simulink model "p2"  (R2021a)
settings: Solver=FixedStepAuto  StartTime=0.0  StopTime=inf  RelTol=1e-3
settings Model: EnablePacing=on  Creator=Abbas  LastModifiedBy=smrh1

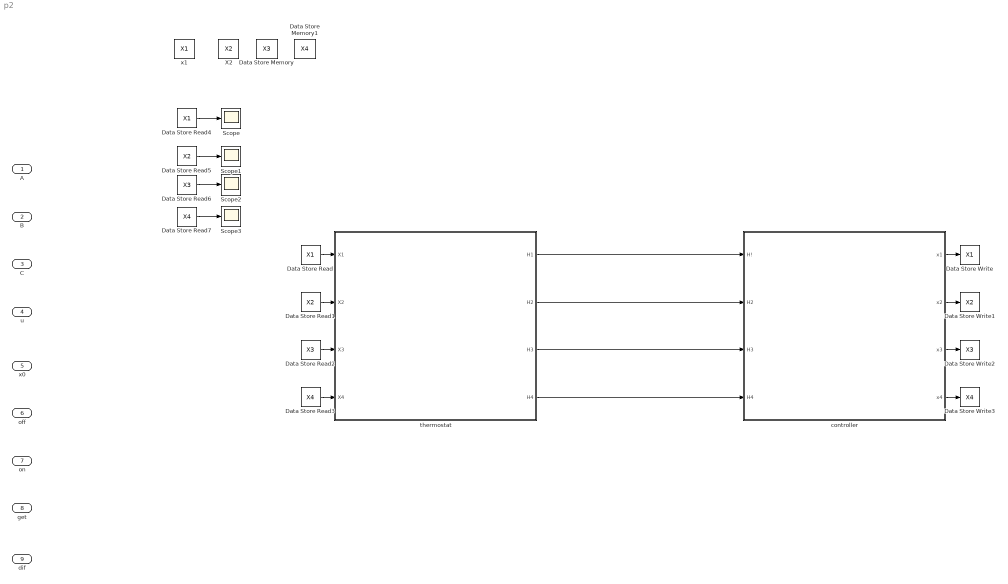
== system p2 ==
  A : Inport
  B : Inport  Port=2
  C : Inport  Port=3
  u : Inport  Port=4
  x0 : Inport  Port=5
  off : Inport  Port=6
  on : Inport  Port=7
  get : Inport  Port=8
  dif : Inport  Port=9
  Data Store Memory : DataStoreMemory  DataStoreName=X3  ReadBeforeWriteMsg=warning  WriteAfterWriteMsg=warning  WriteAfterReadMsg=warning  InitialValue=16.5  ShowAdditionalParam=off
  Data Store Memory1 : DataStoreMemory  DataStoreName=X4  ReadBeforeWriteMsg=warning  WriteAfterWriteMsg=warning  WriteAfterReadMsg=warning  InitialValue=16.5  ShowAdditionalParam=off
  Data Store Read : DataStoreRead  DataStoreName=X1  IndexOptions=Index vector (dialog)  Indices=1  OutputSizes=1
  Data Store Read1 : DataStoreRead  DataStoreName=X2  IndexOptions=Index vector (dialog)  Indices=1  OutputSizes=1
  Data Store Read2 : DataStoreRead  DataStoreName=X3  IndexOptions=Index vector (dialog)  Indices=1  OutputSizes=1
  Data Store Read3 : DataStoreRead  DataStoreName=X4  IndexOptions=Index vector (dialog)  Indices=1  OutputSizes=1
  Data Store Read4 : DataStoreRead  DataStoreName=X1  IndexOptions=Index vector (dialog)  Indices=1  OutputSizes=1
  Data Store Read5 : DataStoreRead  DataStoreName=X2  IndexOptions=Index vector (dialog)  Indices=1  OutputSizes=1
  Data Store Read6 : DataStoreRead  DataStoreName=X3  IndexOptions=Index vector (dialog)  Indices=1  OutputSizes=1
  Data Store Read7 : DataStoreRead  DataStoreName=X4  IndexOptions=Index vector (dialog)  Indices=1  OutputSizes=1
  Data Store Write : DataStoreWrite  DataStoreName=X1  IndexOptions=Index vector (dialog)  Indices=1  OutputSizes=1
  Data Store Write1 : DataStoreWrite  DataStoreName=X2  IndexOptions=Index vector (dialog)  Indices=1  OutputSizes=1
  Data Store Write2 : DataStoreWrite  DataStoreName=X3  IndexOptions=Index vector (dialog)  Indices=1  OutputSizes=1
  Data Store Write3 : DataStoreWrite  DataStoreName=X4  IndexOptions=Index vector (dialog)  Indices=1  OutputSizes=1
  Scope{,1..3} (4 alike) : Scope
  X2 : DataStoreMemory  DataStoreName=X2  ReadBeforeWriteMsg=warning  WriteAfterWriteMsg=warning  WriteAfterReadMsg=warning  InitialValue=16.5  ShowAdditionalParam=off
  controller : Subsystem
  thermostat : Subsystem
  x1 : DataStoreMemory  DataStoreName=X1  ReadBeforeWriteMsg=warning  WriteAfterWriteMsg=warning  WriteAfterReadMsg=warning  InitialValue=16.5  ShowAdditionalParam=off
  wires:
  thermostat/4(H4) -> controller/4(H4)
  thermostat/3(H3) -> controller/3(H3)
  thermostat/2(H2) -> controller/2(H2)
  thermostat/1(H1) -> controller/1(H!)
  controller/1(x1) -> Data Store Write/1
  Data Store Read/1 -> thermostat/1(X1)
  Data Store Read1/1 -> thermostat/2(X2)
  Data Store Read2/1 -> thermostat/3(X3)
  Data Store Read3/1 -> thermostat/4(X4)
  controller/2(x2) -> Data Store Write1/1
  controller/3(x3) -> Data Store Write2/1
  controller/4(x4) -> Data Store Write3/1
  Data Store Read4/1 -> Scope/1
  Data Store Read5/1 -> Scope1/1
  Data Store Read6/1 -> Scope2/1
  Data Store Read7/1 -> Scope3/1

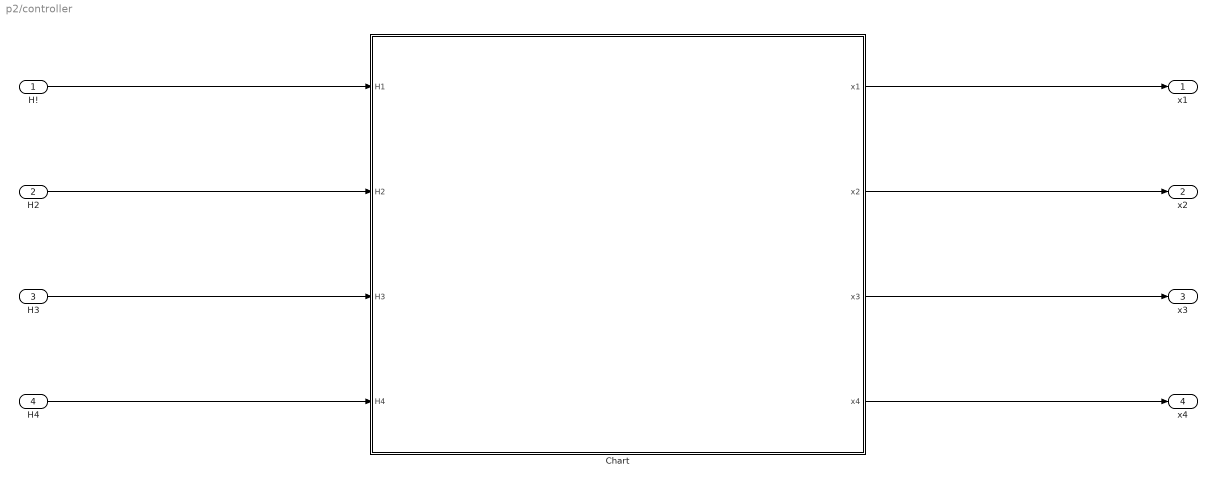
== system p2/controller ==
  H! : Inport
  H2 : Inport  Port=2
  H3 : Inport  Port=3
  H4 : Inport  Port=4
  Chart : Stateflow chart  TreatAsAtomicUnit=on
  x1 : Outport
  x2 : Outport  Port=2
  x3 : Outport  Port=3
  x4 : Outport  Port=4
  wires:
  Chart/1(x1) -> x1/1
  Chart/2(x2) -> x2/1
  Chart/3(x3) -> x3/1
  Chart/4(x4) -> x4/1
  H!/1 -> Chart/1(H1)
  H2/1 -> Chart/2(H2)
  H3/1 -> Chart/3(H3)
  H4/1 -> Chart/4(H4)

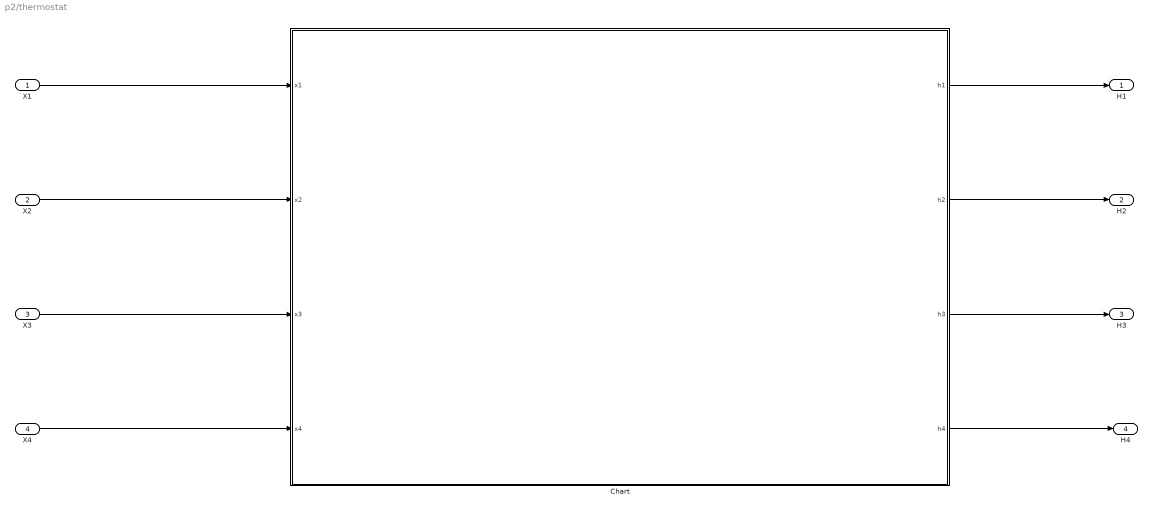
== system p2/thermostat ==
  X1 : Inport
  X2 : Inport  Port=2
  X3 : Inport  Port=3
  X4 : Inport  Port=4
  Chart : Stateflow chart  TreatAsAtomicUnit=on
  H1 : Outport
  H2 : Outport  Port=2
  H3 : Outport  Port=3
  H4 : Outport  Port=4
  wires:
  Chart/1(h1) -> H1/1
  Chart/2(h2) -> H2/1
  Chart/3(h3) -> H3/1
  Chart/4(h4) -> H4/1
  X2/1 -> Chart/2(x2)
  X4/1 -> Chart/4(x4)
  X3/1 -> Chart/3(x3)
  X1/1 -> Chart/1(x1)

== stateflow chart p2/thermostat/Chart ==
  state st13
    du:
    h2 = 0;
    h4 = 0;
    state s1 [parallel]
      settings: executionOrder=1
      state s1_on
        du:
        h1 = 1
      state s1_off
        du:
        h1 = 0
      st13.s1.s1_on -> ? : [x1>=off1& after(1,sec)]
      st13.s1.s1_off -> st13.s1.s1_on : [x1<=on1& after(1,sec)]
      (default) -> st13.s1.s1_off
    state s2 [parallel]
      settings: executionOrder=2
      state s3_on
        du:
        h3 = 1
      state s3_off
        du:
        h3 = 0
      st13.s2.s3_on -> ? : [x3>=off3& after(1,sec)]
      st13.s2.s3_off -> st13.s2.s3_on : [x3<=on3& after(1,sec)]
      (default) -> st13.s2.s3_off
  state st14
    du:
    h2 = 0;
    h3 = 0;
    state s1 [parallel]
      settings: executionOrder=1
      state s1_on
        du:
        h1 = 1
      state s1_off
        du:
        h1 = 0
      st14.s1.s1_on -> ? : [x1>=off1& after(1,sec)]
      st14.s1.s1_off -> st14.s1.s1_on : [x1<=on1& after(1,sec)]
      (default) -> st14.s1.s1_off
    state s4 [parallel]
      settings: executionOrder=2
      state s4_on
        du:
        h4 = 1
      state s4_off
        du:
        h4 = 0
      st14.s4.s4_on -> ? : [x4>=off4& after(1,sec)]
      st14.s4.s4_off -> st14.s4.s4_on : [x4<=on4& after(1,sec)]
      (default) -> st14.s4.s4_off
  state st12
    du:
    h3 = 0;
    h4 = 0;
    state s1 [parallel]
      settings: executionOrder=1
      state s1_on1
        du:
        h1 = 1
      state s1_off
        du:
        h1 = 0
      s1_on1 -> ? : [x1>=off1 & after(1,sec)]
      st12.s1.s1_off -> s1_on1 : [x1<=on1 & after(1,sec)]
      (default) -> st12.s1.s1_off
    state s2 [parallel]
      settings: executionOrder=2
      state s2_on
        du:
        h2 = 1
      state s1_off1
        du:
        h2 = 0
      st12.s2.s2_on -> ? : [x2>=off2 & after(1,sec)]
      s1_off1 -> st12.s2.s2_on : [x2<=on2 & after(1,sec)]
      (default) -> s1_off1
  state st24
    du:
    h1 = 0;
    h3 = 0;
    state s2 [parallel]
      settings: executionOrder=1
      state s2_on
        du:
        h2 = 1
      state s2_off
        du:
        h2 = 0
      st24.s2.s2_on -> ? : [x2>=off2& after(1,sec)]
      s2_off -> st24.s2.s2_on : [x2<=on2& after(1,sec)]
      (default) -> s2_off
    state s4 [parallel]
      settings: executionOrder=2
      state s4_on
        du:
        h4 = 1
      state s4_off
        du:
        h4 = 0
      st24.s4.s4_on -> ? : [x4>=off4& after(1,sec)]
      st24.s4.s4_off -> st24.s4.s4_on : [x4<=on4& after(1,sec)]
      (default) -> st24.s4.s4_off
  state st34
    du:
    h1 = 0;
    h2 = 0;
    state s3 [parallel]
      settings: executionOrder=1
      state s3_on
        du:
        h3 = 1
      state s3_off
        du:
        h3 = 0
      st34.s3.s3_on -> ? : [x1>=off1& after(1,sec)]
      st34.s3.s3_off -> st34.s3.s3_on : [x1<=on1& after(1,sec)]
      (default) -> st34.s3.s3_off
    state s4 [parallel]
      settings: executionOrder=2
      state s4_on
        du:
        h4 = 1
      state s4_off
        du:
        h4 = 0
      st34.s4.s4_on -> ? : [x4>=off4& after(1,sec)]
      st34.s4.s4_off -> st34.s4.s4_on : [x4<=on4& after(1,sec)]
      (default) -> st34.s4.s4_off
  state st23
    du:
    h1 = 0;
    h4 = 0;
    state s2 [parallel]
      settings: executionOrder=1
      state s2_on
        du:
        h2 = 1
      state s1_off
        du:
        h2 = 0
      (default) -> st23.s2.s2_on
      st23.s2.s2_on -> ? : [x2>=off2 & after(1,sec)]
      st23.s2.s1_off -> st23.s2.s2_on : [x2<=on2& after(1,sec)]
    state s3 [parallel]
      settings: executionOrder=2
      state s3_on
        du:
        h3 = 1
      state s3_off
        du:
        h3 = 0
      (default) -> st23.s3.s3_on
      st23.s3.s3_on -> ? : [x3>=off3& after(1,sec)]
      st23.s3.s3_off -> st23.s3.s3_on : [x3<=on3 & after(1,sec)]
  state start
  st12 -> st13 [order 1] : [x2-x3>=dif3 & x3<=get3]
  st13 -> st14 [order 2] : [x3-x4>=dif4 & x4<=get4]
  st13 -> st12 [order 1] : [x3-x2>=dif2 & x2<=get2]
  st14 -> st13 [order 2] : [x4-x3>=dif3 & x3<=get3]
  st13 -> st34 [order 5] : [x1-x4>=dif4 & x4<=get4]
  st34 -> st13 [order 2] : [x4-x1>=dif1 & x1<=get1]
  st13 -> st23 [order 3] : [(x1-x2>=dif2 & x2<=get2)]
  st23 -> st14 [order 3] : [((x2-x4>=dif4 & x4<=get4) & (x3-x1>=dif1 & x1<=get1)) | ((x3-x4>=dif4 & x4<=get4) & (x2-x1>=dif1 & x1<=get1))]
  st23 -> st13 [order 2] : [(x2-x1>=dif1 & x1<=get1)]
  st14 -> st23 [order 3] : [((x4-x2>=dif2 & x2<=get2) & (x1-x3>=dif3 & x3<=get3)) |((x1-x2>=dif2 & x2<=get2) & (x4-x3>=dif3 & x3<=get3))]
  st12 -> st14 [order 3] : [x2-x4>=dif4 & x4<=get4]
  st14 -> st12 [order 1] : [x4-x2>=dif2 & x2<=get2]
  st12 -> st34 [order 5] : [((x1-x4>=dif4 & x4<=get4) & (x2-x3>=dif3 & x3<=get3)) | ((x2-x4>=dif4 & x4<=get4) & (x1-x3>=dif3 & x3<=get3))]
  st34 -> st12 [order 1] : [((x4-x1>=dif1 & x1<=get1) & (x3-x2>=dif2 & x2<=get2)) | ((x2-x4>=dif4 & x4<=get4) & (x1-x3>=dif3 & x3<=get3))]
  st14 -> st34 [order 5] : [x1-x3>=dif3 & x3<=get3]
  st34 -> st14 [order 3] : [x3-x1>=dif1 & x1<=get1]
  st13 -> st24 [order 4] : [((x1-x2>=dif2 & x2<=get2) & (x3-x4>=dif4 & x4<=get4)) | ((x3-x2>=dif2 & x2<=get2) & (x1-x4>=dif4 & x4<=get4))]
  st24 -> st13 [order 2] : [((x2-x1>=dif1 & x1<=get1) & (x4-x3>=dif3 & x3<=get3)) | ((x4-x1>=dif1 & x1<=get1) & (x2-x3>=dif3 & x3<=get3))]
  st24 -> st14 [order 3] : [x2-x4>=dif4 & x4<=get4]
  st14 -> st24 [order 4] : [x4-x2>=dif2 & x2<=get2]
  st12 -> st23 [order 2] : [x1-x3>=dif3 & x3<=get3]
  st23 -> st12 [order 1] : [x3-x1>=dif1 & x1<=get1]
  st24 -> st12 [order 1] : [x4-x1>=dif1 & x1<=get1]
  st12 -> st24 [order 4] : [x1-x4>=dif4 & x4<=get4]
  (default) -> start
  start -> st23 : [true]
  st23 -> st24 [order 4] : [x3-x4>=dif4 & x4<=get4]
  st24 -> st34 [order 5] : [x2-x3>=dif3 & x3<=get3]
  st24 -> st23 [order 4] : [x4-x3>=dif3 & x3<=get3]
  st34 -> st24 [order 5] : [x3-x2>=dif2 & x2<=get2]
  st23 -> st34 [order 5] : [x2-x4>=dif4 & x4<=get4]
  st34 -> st23 [order 4] : [x4-x2>=dif2 & x2<=get2]
  data: on1 local double =19; on2 local double =19; on3 local double =19; on4 local double =19; off1 local double =20; off2 local double =20; off3 local double =20; off4 local double =20; get1 local double =17; get2 local double =16; get3 local double =16; get4 local double =17; dif1 local double =1; dif2 local double =1; dif3 local double =1; dif4 local double =1; x1 input double; x2 input double; x3 input double; h1 output double; h2 output double; h3 output double; h4 output double; x01 local double =16.5; x02 local double =16.5; x03 local double =16.5; x04 local double =16.5; x4 input double

== stateflow chart p2/controller/Chart ==
  settings: updateMethod=CONTINUOUS
  state state_1
    du:
    x1_dot = H1*C1 + B1*(u-x1)+A12*(x1-x2) + A13*(x1-x3) + A14*(x1-x4);
    x2_dot = H2*C2 + B2*(u-x2)+A21*(x2-x1) + A23*(x2-x3) + A24*(x2-x4);
    x3_dot = H3*C3 + B3*(u-x3)+A31*(x3-x1) + A32*(x3-x2) + A34*(x3-x4);
    x4_dot = H4*C4 + B4*(u-x4)+A41*(x4-x1) + A42*(x4-x2) + A43*(x4-x3);
  (default) -> state_1 : {x1 = x01; x2 = x02;x3 = x03;x4 = x04;}
  data: A12 local =0.3; A13 local =0.4; A14 local =0.3; A21 local =0.3; A23 local =0.5; A24 local =0; A31 local =0.4; A32 local =0.5; A34 local =0.3; A41 local =0.3; A42 local =0; A43 local =0.3; B1 local =0.3; B2 local =0.2; B3 local =0.5; B4 local =0.4; C1 local =9; C2 local =7; C3 local =11; C4 local =7; x01 local =16.5; x02 local =16.5; x03 local =16.5; x04 local =16.5; u local =6; H1 input =0; H2 input =1; H3 input =0; H4 input =1; x1 output; x2 output; x3 output; x4 output
  data x1 settings: updateMethod=SF_CONTINUOUS_TIME_DATA
  data x2 settings: updateMethod=SF_CONTINUOUS_TIME_DATA
  data x3 settings: updateMethod=SF_CONTINUOUS_TIME_DATA
  data x4 settings: updateMethod=SF_CONTINUOUS_TIME_DATA
